simulink model "PWM_model"  (R2024a)
settings: Solver=odeN  StartTime=0.0  StopTime=35  MaxStep=5e-05  RelTol=0.001  EnableMultiTasking=on
InitFcn:
  | load bldcData
model workspace (MAT data in the model file):
  encoderResolution = 2000
  hallOffset = '0.5'
  indexOffset = 850
  polePairs = '4'
undefined symbols (not defined in the file or in its folder): DiscIntNeverNeededParam, Hecate_speed, Ts_motor
libraries: nesl_utility x20, fl_lib x18, ee_lib x10, spsPWMGeneratorDCDCLib x2, slpidlib x2, batteryecm_lib x1, simulink x1
(part 2 of 2)

== stateflow chart PWM_model/Test Sequence speed ==
  state Grafico_Scalino_1
    state step_1
      speed = 0;
    state step_2
      speed = Hecate_speed;
    (default) -> Grafico_Scalino_1.step_1
    Grafico_Scalino_1.step_1 -> Grafico_Scalino_1.step_2 : [
        | after(1,'sec')
        | ]
    Grafico_Scalino_1.step_2 -> Grafico_Scalino_1.step_1 : [
        | after(4,'sec')
        | ]
  state Grafico_Scalino_2
    state step_1
      speed = 85;
    state step_2
      speed = Hecate_speed;
    (default) -> Grafico_Scalino_2.step_1
    Grafico_Scalino_2.step_1 -> Grafico_Scalino_2.step_2 : [
        | after(1,'sec')
        | ]
    Grafico_Scalino_2.step_2 -> Grafico_Scalino_2.step_1 : [
        | after(4,'sec')
        | ]
  state Grafico_Scalino_3
    state step_1
      speed = 130;
    state step_2
      speed = Hecate_speed;
    (default) -> Grafico_Scalino_3.step_1
    Grafico_Scalino_3.step_1 -> Grafico_Scalino_3.step_2 : [
        | after(1,'sec')
        | ]
    Grafico_Scalino_3.step_2 -> Grafico_Scalino_3.step_1 : [
        | after(4,'sec')
        | ]
  state Grafico_DoppioTronco_1
    state step_1
      getSimulationTime()
      speed = 0 + (Hecate_speed - 0) / (5 - 0) * getSimulationTime();
    state step_2
      speed = Hecate_speed;
    state step_3
      speed = Hecate_speed + (0 - Hecate_speed) / (15 - 10) * (getSimulationTime - 10);
    state step_4
      speed = 0;
    state step_5
      speed = 0 + (Hecate_speed - 0) / (5 - 0) * (getSimulationTime() - 20);
    state step_6
      speed = Hecate_speed;
    state step_7
      speed = Hecate_speed + (0 - Hecate_speed) / (15 - 10) * (getSimulationTime - 30);
    (default) -> Grafico_DoppioTronco_1.step_1
    Grafico_DoppioTronco_1.step_1 -> Grafico_DoppioTronco_1.step_2 : [
        | after(5, 'sec')
        | ]
    Grafico_DoppioTronco_1.step_2 -> Grafico_DoppioTronco_1.step_3 : [
        | after(5, 'sec')
        | ]
    Grafico_DoppioTronco_1.step_3 -> Grafico_DoppioTronco_1.step_4 : [
        | after(5, 'sec')
        | ]
    Grafico_DoppioTronco_1.step_4 -> Grafico_DoppioTronco_1.step_5 : [
        | after(5, 'sec')
        | ]
    Grafico_DoppioTronco_1.step_5 -> Grafico_DoppioTronco_1.step_6 : [
        | after(5, 'sec')
        | ]
    Grafico_DoppioTronco_1.step_6 -> Grafico_DoppioTronco_1.step_7 : [
        | after(5, 'sec')
        | ]
  state Grafico_DoppioTronco_2
    state step_1
      getSimulationTime()
      speed = 85 + (Hecate_speed - 85) / (5 - 0) * getSimulationTime();
    state step_2
      speed = Hecate_speed;
    state step_3
      speed = Hecate_speed + (85 - Hecate_speed) / (15 - 10) * (getSimulationTime - 10);
    state step_4
      speed = 85;
    state step_5
      speed = 85 + (Hecate_speed - 85) / (5 - 0) * (getSimulationTime() - 20);
    state step_6
      speed = Hecate_speed;
    state step_7
      speed = Hecate_speed + (85 - Hecate_speed) / (15 - 10) * (getSimulationTime - 30);
    (default) -> Grafico_DoppioTronco_2.step_1
    Grafico_DoppioTronco_2.step_1 -> Grafico_DoppioTronco_2.step_2 : [
        | after(5, 'sec')
        | ]
    Grafico_DoppioTronco_2.step_2 -> Grafico_DoppioTronco_2.step_3 : [
        | after(5, 'sec')
        | ]
    Grafico_DoppioTronco_2.step_3 -> Grafico_DoppioTronco_2.step_4 : [
        | after(5, 'sec')
        | ]
    Grafico_DoppioTronco_2.step_4 -> Grafico_DoppioTronco_2.step_5 : [
        | after(5, 'sec')
        | ]
    Grafico_DoppioTronco_2.step_5 -> Grafico_DoppioTronco_2.step_6 : [
        | after(5, 'sec')
        | ]
    Grafico_DoppioTronco_2.step_6 -> Grafico_DoppioTronco_2.step_7 : [
        | after(5, 'sec')
        | ]
  state Grafico_DoppioTronco_3
    state step_1
      getSimulationTime()
      speed = 130 + (Hecate_speed - 130) / (5 - 0) * getSimulationTime();
    state step_2
      speed = Hecate_speed;
    state step_3
      speed = Hecate_speed + (130 - Hecate_speed) / (15 - 10) * (getSimulationTime - 10);
    state step_4
      speed = 130;
    state step_5
      speed = 130 + (Hecate_speed - 130) / (5 - 0) * (getSimulationTime() - 20);
    state step_6
      speed = Hecate_speed;
    state step_7
      speed = Hecate_speed + (130 - Hecate_speed) / (15 - 10) * (getSimulationTime - 30);
    (default) -> Grafico_DoppioTronco_3.step_1
    Grafico_DoppioTronco_3.step_1 -> Grafico_DoppioTronco_3.step_2 : [
        | after(5, 'sec')
        | ]
    Grafico_DoppioTronco_3.step_2 -> Grafico_DoppioTronco_3.step_3 : [
        | after(5, 'sec')
        | ]
    Grafico_DoppioTronco_3.step_3 -> Grafico_DoppioTronco_3.step_4 : [
        | after(5, 'sec')
        | ]
    Grafico_DoppioTronco_3.step_4 -> Grafico_DoppioTronco_3.step_5 : [
        | after(5, 'sec')
        | ]
    Grafico_DoppioTronco_3.step_5 -> Grafico_DoppioTronco_3.step_6 : [
        | after(5, 'sec')
        | ]
    Grafico_DoppioTronco_3.step_6 -> Grafico_DoppioTronco_3.step_7 : [
        | after(5, 'sec')
        | ]
  (default) -> Grafico_Scalino_1 [order 1] : [Active_Scenario_Index == 1]
  (default) -> Grafico_Scalino_2 [order 2] : [Active_Scenario_Index == 2]
  (default) -> Grafico_Scalino_3 [order 3] : [Active_Scenario_Index == 3]
  (default) -> Grafico_DoppioTronco_1 [order 4] : [Active_Scenario_Index == 4]
  (default) -> Grafico_DoppioTronco_2 [order 5] : [Active_Scenario_Index == 5]
  (default) -> Grafico_DoppioTronco_3 [order 6] : {assert(Active_Scenario_Index == 6,'The value of Scenario Parameter ''Active_Scenario_Index'' is not valid. Use the index of the scenario to specify it.')}
  data: speed output; Active_Scenario_Index parameter =1; Hecate_speed parameter

== stateflow chart PWM_model/FitnessConverter_Hecate ==
  state step_1
    fitness_1 = Inf;
  state step_2
    fitness_1 = (Hecate_speed+1)-(speed);
  (default) -> step_1
  step_2 -> step_1 : [after(4, 'sec')]
  step_1 -> step_2 : [after(26, 'sec')]
  data: voltage input; current input; speed input; acc input; Hecate_speed parameter; fitness_1 output

== stateflow chart PWM_model/Test Assessment ==
  state SpeedLimit_0
    state step_1
    state step_2
      verify(speed >= 0.0001);
    (default) -> SpeedLimit_0.step_1
    SpeedLimit_0.step_1 -> step_2 : [
        | after(2, 'sec')
        | ]
  state SpeedLimit_170
    state Speed_Hecate
      verify(speed <=  170);
    (default) -> SpeedLimit_170.Speed_Hecate
  state SpeedLimit_HS
    state step_1
      % Initial and Final Waiting Period
    state Speed_Hecate
      verify(speed <= (Hecate_speed + 1));
    state step_3
      % Midpoint Waiting Period
    state Speed_Hecate_1
      verify(speed <= (Hecate_speed + 1));
    (default) -> SpeedLimit_HS.step_1
    (junction 384) -> SpeedLimit_HS.step_1
    SpeedLimit_HS.step_1 -> SpeedLimit_HS.Speed_Hecate : [
        | after(6, 'sec')
        | ]
    SpeedLimit_HS.Speed_Hecate -> step_3 : [
        | after(4, 'sec')
        | ]
    step_3 -> Speed_Hecate_1 : [
        | after(16, 'sec')
        | ]
    Speed_Hecate_1 -> (junction 386) : [
        | after(4, 'sec')
        | ]
    (junction 386) -> (junction 384)
  state SpeedLimit_HS_subtest
    state step_1
    state Speed_Hecate
      verify(speed <= (Hecate_speed + 1));
    (default) -> SpeedLimit_HS_subtest.step_1
    SpeedLimit_HS_subtest.step_1 -> SpeedLimit_HS_subtest.Speed_Hecate : [
        | after(26, 'sec')
        | ]
    SpeedLimit_HS_subtest.Speed_Hecate -> SpeedLimit_HS_subtest.step_1 : [
        | after(4, 'sec')
        | ]
  (default) -> SpeedLimit_0 [order 1] : [Active_Scenario_Index == 1]
  (default) -> SpeedLimit_170 [order 2] : [Active_Scenario_Index == 2]
  (default) -> SpeedLimit_HS [order 3] : [Active_Scenario_Index == 3]
  (default) -> SpeedLimit_HS_subtest [order 4] : {assert(Active_Scenario_Index == 4,'The value of Scenario Parameter ''Active_Scenario_Index'' is not valid. Use the index of the scenario to specify it.')}
  data: voltage input; current input; speed input; acc input; Active_Scenario_Index parameter =1; speed_at_5_5 local; speed_at_9 local; Hecate_speed parameter
